simulink model "test2"  (R2024a)
settings: Solver=VariableStepAuto  StartTime=0.0  StopTime=1000  RelTol=1e-3
undefined symbols (not defined in the file or in its folder): ref, x
libraries: simulink x1
settings Model: Creator=b_ant  LastModifiedBy=b_ant

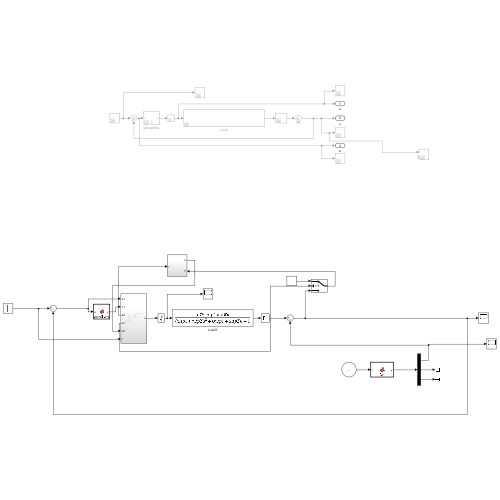
[thumbnail: Simulink's stored preview of the top-level diagram]
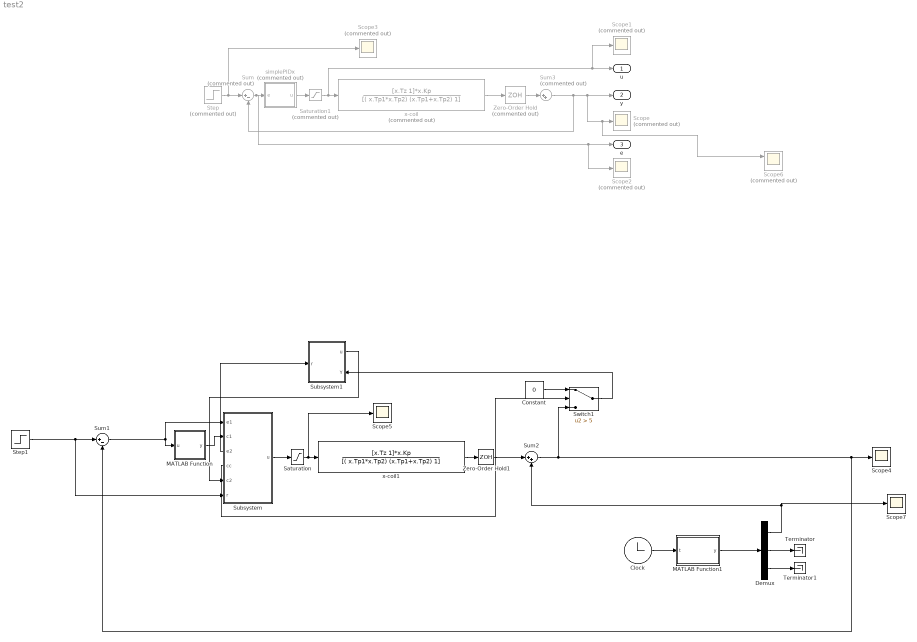
== system test2 ==
  Clock : Clock
  Constant : Constant  Value=0
  Demux : Demux  Outputs=3
  MATLAB Function : MATLAB Function  TreatAsAtomicUnit=on
  MATLAB Function1 : MATLAB Function  TreatAsAtomicUnit=on
  Saturation : Saturate  UpperLimit=15  LowerLimit=-15
  Saturation1 : Saturate  Commented=on  UpperLimit=15  LowerLimit=-15
  Scope{,1..3} (4 alike) : Scope  Commented=on
  Scope4 : Scope
  Scope5 : Scope
  Scope6 : Scope  Commented=on  NumInputPorts=2
  Scope7 : Scope
  Step : Step  Commented=on  Time=0.0001  SampleTime=0
  Step1 : Step  Time=0.0001  SampleTime=0
  Subsystem : Subsystem
      settings: PortSchema="{\"entries\":[{\"content\":{\"sides\":[{\"content\":{\"connectorIds\":[\"In1\",\"In2\",\"Out2\",\"Out3\",\"In3\",\"In4\"]},\"type\":\"ConnectorPlacement.EquallySpacedRectSide\",\"uuid\":\"7068f7a8-39a5-4b81-9242-0ff684ad2d52\"},{\"content\":{\"connectorIds\":[\"Out1\"],\"side\":\"RIGHT\"},\"type\":\"ConnectorPlacement.EquallySpacedRectSide\",\"uuid\":\"6f619d2f-5996-4772-917a-a91f12c99af0\"},{\"content\":{\"side\":\"TOP\"},\"type\":\"ConnectorPlacement.EquallySpacedRectSide\",\"uuid\":\"a18f3392-cfd4-4b10-bccf-639e40fe0ff5\"}]},\"type\":\"ConnectorPlacement.EquallySpacedConnector\",\"uuid\":\"3030bedd-17ea-4c41-8905-7d24d55e9816\"}],\"packageUris\":[\"http://schema.mathworks.com/mf0/Connector/R2020b\"],\"version\":\"1.0\"}"
  Subsystem1 : Subsystem
      settings: PortSchema="{\"entries\":[{\"content\":{\"sides\":[{\"content\":{\"connectorIds\":[\"In1\"]},\"type\":\"ConnectorPlacement.EquallySpacedRectSide\",\"uuid\":\"1b9826ce-63ba-49e6-baba-5607636d1395\"},{\"content\":{\"connectorIds\":[\"Out1\",\"In2\"],\"side\":\"RIGHT\"},\"type\":\"ConnectorPlacement.EquallySpacedRectSide\",\"uuid\":\"62ed80bc-b8a6-45eb-884b-60ca6a43fc6d\"},{\"content\":{\"side\":\"TOP\"},\"type\":\"ConnectorPlacement.EquallySpacedRectSide\",\"uuid\":\"dfa23841-0873-4e34-9953-9a9fa94c4c73\"}]},\"type\":\"ConnectorPlacement.EquallySpacedConnector\",\"uuid\":\"19a1b559-d4d9-41ef-bb40-5c1232dced78\"}],\"packageUris\":[\"http://schema.mathworks.com/mf0/Connector/R2020b\"],\"version\":\"1.0\"}"
  Sum : Sum  Commented=on  Inputs=|+-
  Sum1 : Sum  Inputs=|+-
  Sum2 : Sum  Inputs=|++
  Sum3 : Sum  Commented=on  Inputs=|++
  Switch1 : Switch  Criteria=u2 > Threshold  Threshold=5  SaturateOnIntegerOverflow=off  InputSameDT=off
  Terminator : Terminator
  Terminator1 : Terminator
  Zero-Order Hold : ZeroOrderHold  Commented=on
  Zero-Order Hold1 : ZeroOrderHold  SampleTime=0.5E-3
  simplePIDx : Subsystem  Commented=on  mask{Gain1=x.PID.Kd, Gain2=x.PID.Ki, Gain3=x.PID.Kp}
      mask prompts: Gain1 "kd:"; Gain2 "ki:"; Gain3 "kp:"
      mask TypeOptions Gain1: PID kd/Gain
      mask TypeOptions Gain2: PID ki/Gain
      mask TypeOptions Gain3: PID kp/Gain
  x-coil : TransferFcn  Commented=on  Numerator=[x.Tz 1]*x.Kp  Denominator=[( x.Tp1*x.Tp2) (x.Tp1+x.Tp2) 1]
  x-coil1 : TransferFcn  Numerator=[x.Tz 1]*x.Kp  Denominator=[( x.Tp1*x.Tp2) (x.Tp1+x.Tp2) 1]
  u : Outport
  y : Outport  Port=2
  e : Outport  Port=3
  wires:
  MATLAB Function/1(y) -> Subsystem/2(c1)
  Clock/1 -> MATLAB Function1/1(t)
  Sum3/1 -> Sum/2, Scope6/1, Scope/1, y/1
  Zero-Order Hold/1 -> Sum3/1
  Demux/1 -> Scope7/1, Sum2/2
  MATLAB Function1/1(y) -> Demux/1
  Demux/2 -> Terminator/1
  Saturation1/1 -> Scope1/1, u/1, x-coil/1
  Step1/1 -> Subsystem/4(r), Sum1/1
  simplePIDx/1(u) -> Saturation1/1
  x-coil/1 -> Zero-Order Hold/1
  Step/1 -> Scope3/1, Sum/1
  Sum/1 -> Scope2/1, e/1, simplePIDx/1(e)
  Subsystem/1(u) -> Saturation/1
  Demux/3 -> Terminator1/1
  Sum1/1 -> Subsystem/1(e1), MATLAB Function/1(u)
  x-coil1/1 -> Zero-Order Hold1/1
  Subsystem1/1(u) -> Subsystem/3(c2)
  Subsystem/2(e2) -> Subsystem1/1(r)
  Subsystem/3(cc) -> Switch1/2
  Sum2/1 -> Switch1/3, Sum1/2, Scope4/1
  Switch1/1 -> Subsystem1/2(Y)
  Constant/1 -> Switch1/1
  Zero-Order Hold1/1 -> Sum2/1
  Saturation/1 -> Scope5/1, x-coil1/1

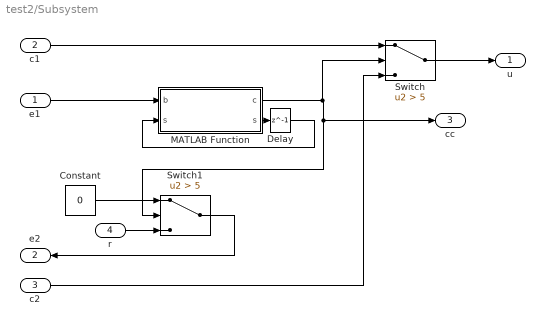
== system test2/Subsystem ==
  e1 : Inport
  c1 : Inport  Port=2
  c2 : Inport  Port=3
  r : Inport  Port=4
  Constant : Constant  Value=0
  Delay : Delay  DelayLength=1
  MATLAB Function : MATLAB Function  TreatAsAtomicUnit=on
  Switch : Switch  Criteria=u2 > Threshold  Threshold=5  SaturateOnIntegerOverflow=off  InputSameDT=off
  Switch1 : Switch  Criteria=u2 > Threshold  Threshold=5  SaturateOnIntegerOverflow=off  InputSameDT=off
  u : Outport
  e2 : Outport  Port=2
  cc : Outport  Port=3
  wires:
  e1/1 -> MATLAB Function/1(b)
  MATLAB Function/2(s) -> Delay/1
  MATLAB Function/1(c) -> Switch/2, cc/1, Switch1/2
  Switch1/1 -> e2/1
  Constant/1 -> Switch1/1
  c1/1 -> Switch/1
  Delay/1 -> MATLAB Function/2("s ")
  Switch/1 -> u/1
  c2/1 -> Switch/3
  r/1 -> Switch1/3

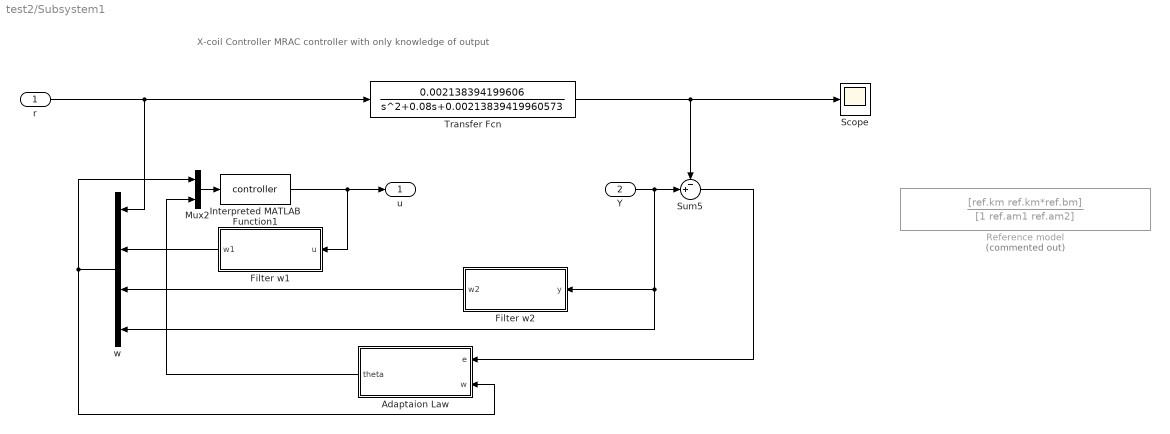
== system test2/Subsystem1 ==
  note: X-coil Controller MRAC controller with only knowledge of output
  r : Inport
  Y : Inport  Port=2
  Adaptaion Law : Subsystem
  Filter w1 : Subsystem
  Filter w2 : Subsystem
  Interpreted MATLAB Function1 : MATLABFcn  MATLABFcn=controller  OutputDimensions=1
  Mux2 : Mux  Inputs=2
  Reference model : TransferFcn  Commented=on  Numerator=[ref.km ref.km*ref.bm]  Denominator=[1 ref.am1 ref.am2]
  Scope : Scope
  Sum5 : Sum  Inputs=-+|
  Transfer Fcn : TransferFcn  Numerator=0.002138394199606  Denominator=[1 0.08 0.00213839419960573]
  w : Mux
  u : Outport
  wires:
  Adaptaion Law/1(theta) -> Mux2/2
  Mux2/1 -> Interpreted MATLAB Function1/1
  Interpreted MATLAB Function1/1 -> u/1, Filter w1/1(u)
  Transfer Fcn/1 -> Sum5/1, Scope/1
  r/1 -> Transfer Fcn/1, w/1
  Y/1 -> Sum5/2, Filter w2/1(y), w/4
  w/1 -> Mux2/1, Adaptaion Law/2(w)
  Filter w1/1(w1) -> w/2
  Sum5/1 -> Adaptaion Law/1(e)
  Filter w2/1(w2) -> w/3

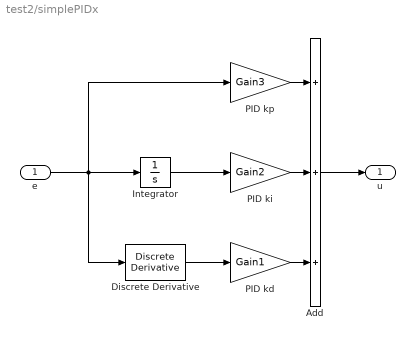
== system test2/simplePIDx ==
  e : Inport
  Add : Sum  Inputs=+++
  Discrete Derivative : simulink/Discrete/Discrete Derivative  gainval=1.0  ICPrevScaledInput=0.0  OutMin=[]  OutMax=[]  OutDataType=fixdt(1, 16)  OutScaling=2^-10  DoSatur=off
  Integrator : Integrator
  PID kd : Gain  Gain=Gain1
  PID ki : Gain  Gain=Gain2
  PID kp : Gain  Gain=Gain3
  u : Outport
  wires:
  Discrete Derivative/1 -> PID kd/1
  Add/1 -> u/1
  e/1 -> PID kp/1, Integrator/1, Discrete Derivative/1
  Integrator/1 -> PID ki/1
  PID ki/1 -> Add/2
  PID kd/1 -> Add/3
  PID kp/1 -> Add/1

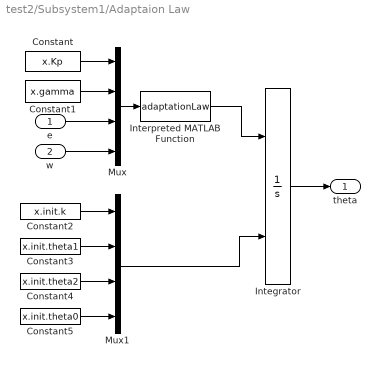
== system test2/Subsystem1/Adaptaion Law ==
  e : Inport
  w : Inport  Port=2
  Constant : Constant  Value=x.Kp
  Constant1 : Constant  Value=x.gamma
  Constant2 : Constant  Value=x.init.k
  Constant3 : Constant  Value=x.init.theta1
  Constant4 : Constant  Value=x.init.theta2
  Constant5 : Constant  Value=x.init.theta0
  Integrator : Integrator  InitialConditionSource=external  InitialCondition=[ref.km/x.Kp,2e-6,2e-6,2e-6]
  Interpreted MATLAB Function : MATLABFcn  MATLABFcn=adaptationLaw  OutputDimensions=4
  Mux : Mux
  Mux1 : Mux
  theta : Outport
  wires:
  Constant1/1 -> Mux/2
  e/1 -> Mux/3
  w/1 -> Mux/4
  Constant/1 -> Mux/1
  Mux/1 -> Interpreted MATLAB Function/1
  Interpreted MATLAB Function/1 -> Integrator/1
  Integrator/1 -> theta/1
  Mux1/1 -> Integrator/2
  Constant2/1 -> Mux1/1
  Constant3/1 -> Mux1/2
  Constant4/1 -> Mux1/3
  Constant5/1 -> Mux1/4

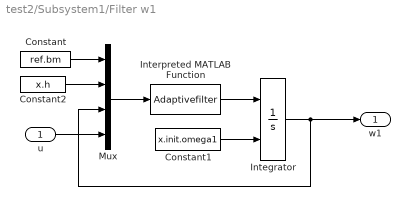
== system test2/Subsystem1/Filter w1 ==
  u : Inport
  Constant : Constant  Value=ref.bm
  Constant1 : Constant  Value=x.init.omega1
  Constant2 : Constant  Value=x.h
  Integrator : Integrator  InitialConditionSource=external  InitialCondition=0.1
  Interpreted MATLAB Function : MATLABFcn  MATLABFcn=Adaptivefilter  OutputDimensions=1
  Mux : Mux
  w1 : Outport
  wires:
  Constant/1 -> Mux/1
  Interpreted MATLAB Function/1 -> Integrator/1
  Mux/1 -> Interpreted MATLAB Function/1
  Integrator/1 -> Mux/3, w1/1
  Constant1/1 -> Integrator/2
  u/1 -> Mux/4
  Constant2/1 -> Mux/2

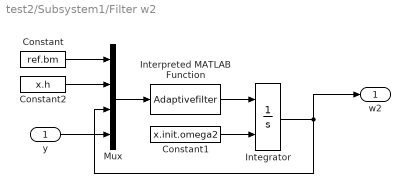
== system test2/Subsystem1/Filter w2 ==
  y : Inport
  Constant : Constant  Value=ref.bm
  Constant1 : Constant  Value=x.init.omega2
  Constant2 : Constant  Value=x.h
  Integrator : Integrator  InitialConditionSource=external  InitialCondition=0.1
  Interpreted MATLAB Function : MATLABFcn  MATLABFcn=Adaptivefilter  OutputDimensions=1
  Mux : Mux
  w2 : Outport
  wires:
  y/1 -> Mux/4
  Constant/1 -> Mux/1
  Interpreted MATLAB Function/1 -> Integrator/1
  Mux/1 -> Interpreted MATLAB Function/1
  Integrator/1 -> Mux/3, w2/1
  Constant1/1 -> Integrator/2
  Constant2/1 -> Mux/2

== matlab function test2/Subsystem/MATLAB Function ==
  data: b input; c output; s input; s output
function [c,s] = selector(b,s)
if(and(or(b >= 0.5, b <= -0.5),s==0))
    c = 10;
else
    c = 0;
    s = 1;
end

== matlab function test2/MATLAB Function ==
  data: u input; y output
function y = bangBang(u)
    y = 15*sign(u);
end

== matlab function test2/MATLAB Function1 ==
  data: t input; y output
function y = fcn(t)
y= [2.522*sin(2*pi*4.788E-3*t)+3.249E04;
   -5.174*sin(2*pi*7.481E-3*t)-2.265E04;
    3.359*sin(2*pi*8.378E-3*t)+3.655E04];
end
